simulink model "zad3_model"  (R2017a)
settings: Solver=VariableStepAuto  StartTime=0.0  StopTime=40  RelTol=1e-3
values from neighbouring files (symbols this model uses):
  K = acker(A2, B2, [z z z])    [zad3a.m]    (also in zad3b.m = acker(A2, B2, [z1 z2 z2]); zad3max.m; zad4.m = acker(Ap, Bp, [0.6 0.4 0.4]))
  Tp = 0.1    [zad3a.m]    (also in zad3b.m; zad3max.m; zad4.m)
settings Model: Creator=Rajtek  LastModifiedBy=Rajtek

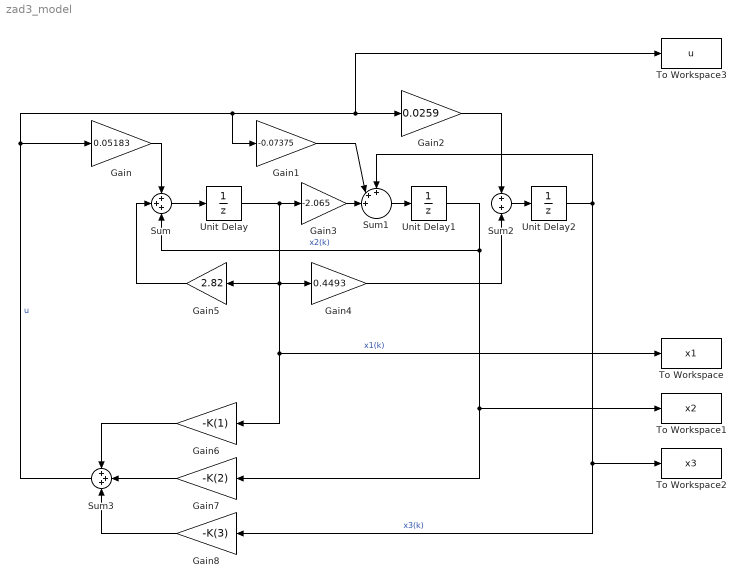
== system zad3_model ==
  Gain : Gain  Gain=0.05183
  Gain1 : Gain  Gain=-0.07375
  Gain2 : Gain  Gain=0.0259
  Gain3 : Gain  Gain=-2.065
  Gain4 : Gain  Gain=0.4493
  Gain5 : Gain  Gain=2.82
  Gain6 : Gain  Gain=-K(1)
  Gain7 : Gain  Gain=-K(2)
  Gain8 : Gain  Gain=-K(3)
  Sum : Sum  Inputs=+++
  Sum1 : Sum  Inputs=+++||
  Sum2 : Sum  Inputs=+|+
  Sum3 : Sum  Inputs=+++
  To Workspace : ToWorkspace  VariableName=x1  SaveFormat=Timeseries  SampleTime=-1
  To Workspace1 : ToWorkspace  VariableName=x2  SaveFormat=Timeseries  SampleTime=-1
  To Workspace2 : ToWorkspace  VariableName=x3  SaveFormat=Timeseries  SampleTime=-1
  To Workspace3 : ToWorkspace  VariableName=u  SaveFormat=Timeseries  SampleTime=-1
  Unit Delay : UnitDelay  InitialCondition=1  SampleTime=Tp
  Unit Delay1 : UnitDelay  InitialCondition=-2  SampleTime=Tp
  Unit Delay2 : UnitDelay  InitialCondition=2  SampleTime=Tp
  wires:
  Unit Delay2/1 -> To Workspace2/1, Gain8/1, Sum1/1  "x3(k)"
  Gain2/1 -> Sum2/1
  Sum3/1 -> Gain/1, To Workspace3/1, Gain2/1, Gain1/1  "u"
  Gain/1 -> Sum/1
  Gain5/1 -> Sum/2
  Gain1/1 -> Sum1/2
  Gain4/1 -> Sum2/2
  Sum2/1 -> Unit Delay2/1
  Unit Delay1/1 -> To Workspace1/1, Gain7/1, Sum/3  "x2(k)"
  Unit Delay/1 -> Gain6/1, To Workspace/1, Gain4/1, Gain5/1, Gain3/1  "x1(k)"
  Gain3/1 -> Sum1/3
  Sum1/1 -> Unit Delay1/1
  Gain7/1 -> Sum3/2
  Gain6/1 -> Sum3/1
  Gain8/1 -> Sum3/3
  Sum/1 -> Unit Delay/1
